simulink model "aula2_2015"  (R2016a)
settings: Solver=ode3  StartTime=0.0  StopTime=Tempo  RelTol=1e-3
values from neighbouring files (symbols this model uses):
  wn = M(turma,I)    [init.m]
undefined symbols (not defined in the file or in its folder): PWM, Ts
settings Model: Creator=CBA2016-05  LastModifiedBy=CBA2016-05
settings HardwareCC: ProdWordSize=32  ProdHWDeviceType=Specified

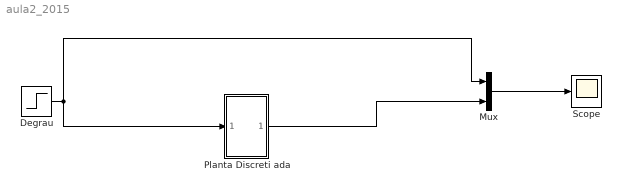
== system aula2_2015 ==
  Degrau : Step  Time=0  After=PWM  SampleTime=0
  Mux : Mux  Inputs=2
  Planta Discreti ada : Subsystem
  Scope : Scope
  wires:
  Mux/1 -> Scope/1
  Degrau/1 -> Planta Discreti ada/1(In1), Mux/1
  Planta Discreti ada/1(Out1) -> Mux/2

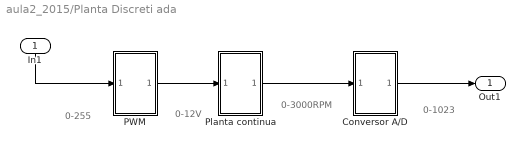
== system aula2_2015/Planta Discreti ada ==
  note: 0-1023
  note: 0-3000RPM
  note: 0-12V
  note: 0-255
  In1 : Inport
  Conversor A/D : Subsystem
  PWM : Subsystem
  Planta continua : Subsystem
  Out1 : Outport
  wires:
  PWM/1(Out1) -> Planta continua/1(In1)
  Conversor A/D/1(Out1) -> Out1/1
  Planta continua/1(Out1) -> Conversor A/D/1(In1)
  In1/1 -> PWM/1(In1)

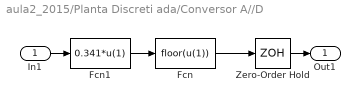
== system aula2_2015/Planta Discreti ada/Conversor A//D ==
  In1 : Inport
  Fcn : Fcn  Expr=floor(u(1))
  Fcn1 : Fcn  Expr=0.341*u(1)
  Zero-Order Hold : ZeroOrderHold  SampleTime=Ts
  Out1 : Outport
  wires:
  Fcn1/1 -> Fcn/1
  Fcn/1 -> Zero-Order Hold/1
  Zero-Order Hold/1 -> Out1/1
  In1/1 -> Fcn1/1

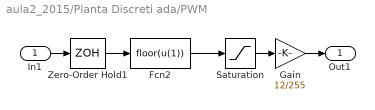
== system aula2_2015/Planta Discreti ada/PWM ==
  In1 : Inport
  Fcn2 : Fcn  Expr=floor(u(1))
  Gain : Gain  Gain=12/255
  Saturation : Saturate  UpperLimit=255  LowerLimit=0
  Zero-Order Hold1 : ZeroOrderHold  SampleTime=Ts
  Out1 : Outport
  wires:
  Zero-Order Hold1/1 -> Fcn2/1
  Saturation/1 -> Gain/1
  Fcn2/1 -> Saturation/1
  Gain/1 -> Out1/1
  In1/1 -> Zero-Order Hold1/1

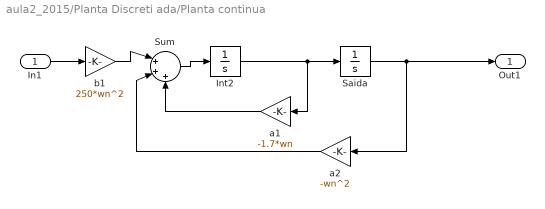
== system aula2_2015/Planta Discreti ada/Planta continua ==
  In1 : Inport
  Int2 : Integrator
  Saida : Integrator
  Sum : Sum  Inputs=|+++
  a1 : Gain  Gain=-1.7*wn
  a2 : Gain  Gain=-wn^2
  b1 : Gain  Gain=250*wn^2
  Out1 : Outport
  wires:
  Sum/1 -> Int2/1
  b1/1 -> Sum/1
  Int2/1 -> a1/1, Saida/1
  a1/1 -> Sum/3
  Saida/1 -> Out1/1, a2/1
  a2/1 -> Sum/2
  In1/1 -> b1/1
